simulink model "dcsim_shelf"  (R2026a)
settings: Solver=ode23t  StopTime=7e-3  MaxStep=1e-6  RelTol=1e-6  AbsTol=1e-6
values from neighbouring files (symbols this model uses):
  prm = [shared.V_ref, shared.P_rated, shared.V_uvlo, c.smooth_on, shared.S_max, shared.tau_r,         shared.p_fix, shared.k2, shared.V_ref48, shared.K_p, shared.K_i, shared.tau_i, shared.I_lim_out,         shared.V_uvlo48, 1.0, shared.t_uvlo48, shared.V_hyst48]    [load_case.m]
undefined symbols (not defined in the file or in its folder): ic_i_co, ic_P_cmd, ic_v_c, ic_v_Cin, ic_v_out, ic_xi_v, R_droop, R_esr, R_f, R_f48, R_in, R_in_esr, R_line, R_out_esr, t_event, tau_c, tau_sense, V_ref
libraries: fl_lib x31, nesl_utility x13
Description:
  | dcsim_shelf build 2026-09-18h (control states integrated explicitly at 1 us in ctrl_d)
settings Model: Creator=USER  LastModifiedBy=USER

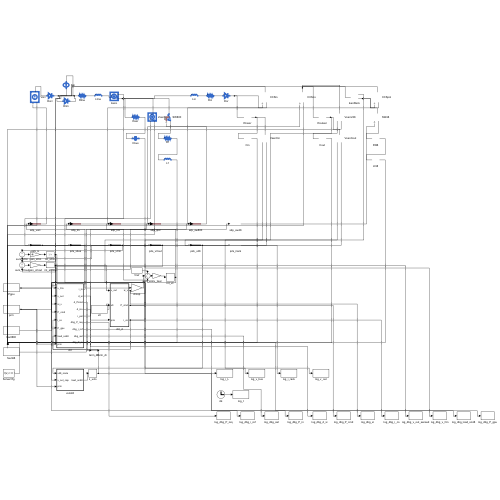
[thumbnail: Simulink's stored preview of the top-level diagram]
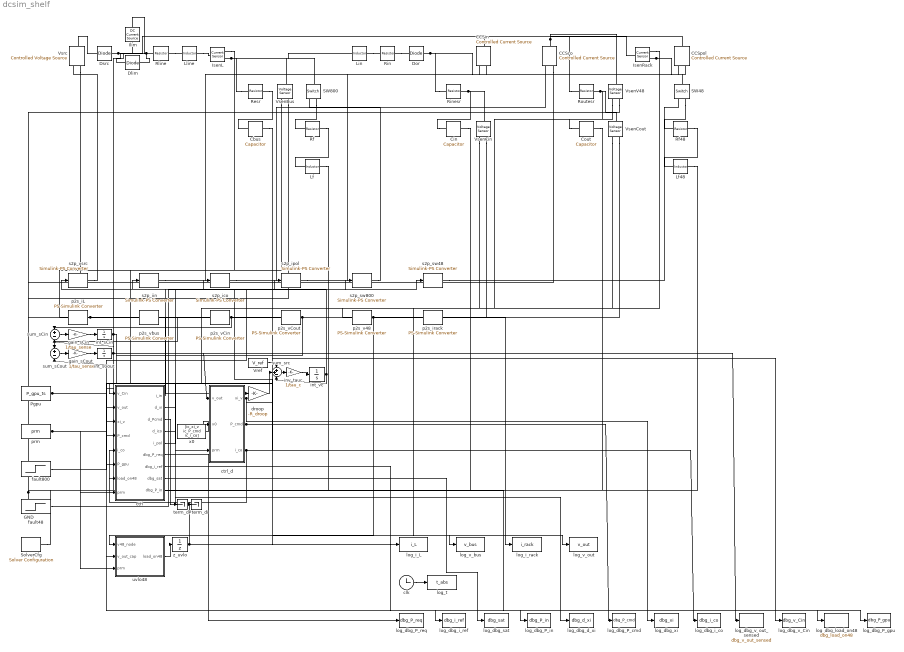
== system dcsim_shelf ==
  CCSco : fl_lib/Electrical/Electrical Sources/Controlled Current Source
  CCSin : fl_lib/Electrical/Electrical Sources/Controlled Current Source
  CCSpol : fl_lib/Electrical/Electrical Sources/Controlled Current Source
  Cbus : fl_lib/Electrical/Electrical Elements/Capacitor  c=C_bus F  r=1e-6 Ohm  g=0 1/Ohm  i_specify=off  i_priority=None  i=0 A  i_nominal_specify=off  i_nominal_value=1  i_nominal_unit=A  v_specify=off  v_priority=None  v=0 V  v_nominal_specify=off  v_nominal_value=1  v_nominal_unit=V  vc_specify=on  vc_priority=High  vc=ic_v_C V  vc_nominal_specify=off  vc_nominal_value=1  vc_nominal_unit=V
  Cin : fl_lib/Electrical/Electrical Elements/Capacitor  c=C_in F  r=1e-6 Ohm  g=0 1/Ohm  i_specify=off  i_priority=None  i=0 A  i_nominal_specify=off  i_nominal_value=1  i_nominal_unit=A  v_specify=off  v_priority=None  v=0 V  v_nominal_specify=off  v_nominal_value=1  v_nominal_unit=V  vc_specify=on  vc_priority=High  vc=ic_v_Cin V  vc_nominal_specify=off  vc_nominal_value=1  vc_nominal_unit=V
  Cout : fl_lib/Electrical/Electrical Elements/Capacitor  c=C_out F  r=1e-6 Ohm  g=0 1/Ohm  i_specify=off  i_priority=None  i=0 A  i_nominal_specify=off  i_nominal_value=1  i_nominal_unit=A  v_specify=off  v_priority=None  v=0 V  v_nominal_specify=off  v_nominal_value=1  v_nominal_unit=V  vc_specify=on  vc_priority=High  vc=ic_v_out V  vc_nominal_specify=off  vc_nominal_value=1  vc_nominal_unit=V
  Dlim : fl_lib/Electrical/Electrical Elements/Diode  Vf=1e-9 V  Ron=1e-6 Ohm  Goff=1e-8 1/Ohm  i_specify=off  i_priority=None  i=0 A  i_nominal_specify=off  i_nominal_value=1  i_nominal_unit=A  v_specify=off  v_priority=None  v=0 V  v_nominal_specify=off  v_nominal_value=1  v_nominal_unit=V
  Dor : fl_lib/Electrical/Electrical Elements/Diode  Vf=1e-9 V  Ron=1e-6 Ohm  Goff=1e-8 1/Ohm  i_specify=off  i_priority=None  i=0 A  i_nominal_specify=off  i_nominal_value=1  i_nominal_unit=A  v_specify=off  v_priority=None  v=0 V  v_nominal_specify=off  v_nominal_value=1  v_nominal_unit=V
  Dsrc : fl_lib/Electrical/Electrical Elements/Diode  Vf=1e-9 V  Ron=1e-6 Ohm  Goff=1e-8 1/Ohm  i_specify=off  i_priority=None  i=0 A  i_nominal_specify=off  i_nominal_value=1  i_nominal_unit=A  v_specify=off  v_priority=None  v=0 V  v_nominal_specify=off  v_nominal_value=1  v_nominal_unit=V
  GND : fl_lib/Electrical/Electrical Elements/Electrical Reference
  Ilim : fl_lib/Electrical/Electrical Sources/DC Current Source  i0=I_lim A
  IsenL : fl_lib/Electrical/Electrical Sensors/Current Sensor
  IsenRack : fl_lib/Electrical/Electrical Sensors/Current Sensor
  Lf : fl_lib/Electrical/Electrical Elements/Inductor  l=L_f H  r=0 Ohm  g=1e-9 1/Ohm  i_specify=off  i_priority=None  i=0 A  i_nominal_specify=off  i_nominal_value=1  i_nominal_unit=A  v_specify=off  v_priority=None  v=0 V  v_nominal_specify=off  v_nominal_value=1  v_nominal_unit=V  i_L_specify=on  i_L_priority=High  i_L=0 A  i_L_nominal_specify=off  i_L_nominal_value=1  i_L_nominal_unit=A
  Lf48 : fl_lib/Electrical/Electrical Elements/Inductor  l=L_f48 H  r=0 Ohm  g=1e-9 1/Ohm  i_specify=off  i_priority=None  i=0 A  i_nominal_specify=off  i_nominal_value=1  i_nominal_unit=A  v_specify=off  v_priority=None  v=0 V  v_nominal_specify=off  v_nominal_value=1  v_nominal_unit=V  i_L_specify=on  i_L_priority=High  i_L=0 A  i_L_nominal_specify=off  i_L_nominal_value=1  i_L_nominal_unit=A
  Lin : fl_lib/Electrical/Electrical Elements/Inductor  l=L_in H  r=0 Ohm  g=1e-9 1/Ohm  i_specify=off  i_priority=None  i=0 A  i_nominal_specify=off  i_nominal_value=1  i_nominal_unit=A  v_specify=off  v_priority=None  v=0 V  v_nominal_specify=off  v_nominal_value=1  v_nominal_unit=V  i_L_specify=on  i_L_priority=High  i_L=ic_i_Lin A  i_L_nominal_specify=off  i_L_nominal_value=1  i_L_nominal_unit=A
  Lline : fl_lib/Electrical/Electrical Elements/Inductor  l=L_line H  r=0 Ohm  g=1e-9 1/Ohm  i_specify=off  i_priority=None  i=0 A  i_nominal_specify=off  i_nominal_value=1  i_nominal_unit=A  v_specify=off  v_priority=None  v=0 V  v_nominal_specify=off  v_nominal_value=1  v_nominal_unit=V  i_L_specify=on  i_L_priority=High  i_L=ic_i_L A  i_L_nominal_specify=off  i_L_nominal_value=1  i_L_nominal_unit=A
  Pgpu : FromWorkspace  VariableName=P_gpu_ts
  Resr : fl_lib/Electrical/Electrical Elements/Resistor  R=R_esr - 1e-6 Ohm  i_specify=off  i_priority=None  i=0 A  i_nominal_specify=off  i_nominal_value=1  i_nominal_unit=A  v_specify=off  v_priority=None  v=0 V  v_nominal_specify=off  v_nominal_value=1  v_nominal_unit=V
  Rf : fl_lib/Electrical/Electrical Elements/Resistor  R=R_f - 1e-6 Ohm  i_specify=off  i_priority=None  i=0 A  i_nominal_specify=off  i_nominal_value=1  i_nominal_unit=A  v_specify=off  v_priority=None  v=0 V  v_nominal_specify=off  v_nominal_value=1  v_nominal_unit=V
  Rf48 : fl_lib/Electrical/Electrical Elements/Resistor  R=R_f48 - 1e-6 Ohm  i_specify=off  i_priority=None  i=0 A  i_nominal_specify=off  i_nominal_value=1  i_nominal_unit=A  v_specify=off  v_priority=None  v=0 V  v_nominal_specify=off  v_nominal_value=1  v_nominal_unit=V
  Rin : fl_lib/Electrical/Electrical Elements/Resistor  R=R_in Ohm  i_specify=off  i_priority=None  i=0 A  i_nominal_specify=off  i_nominal_value=1  i_nominal_unit=A  v_specify=off  v_priority=None  v=0 V  v_nominal_specify=off  v_nominal_value=1  v_nominal_unit=V
  Rinesr : fl_lib/Electrical/Electrical Elements/Resistor  R=R_in_esr - 1e-6 Ohm  i_specify=off  i_priority=None  i=0 A  i_nominal_specify=off  i_nominal_value=1  i_nominal_unit=A  v_specify=off  v_priority=None  v=0 V  v_nominal_specify=off  v_nominal_value=1  v_nominal_unit=V
  Rline : fl_lib/Electrical/Electrical Elements/Resistor  R=R_line Ohm  i_specify=off  i_priority=None  i=0 A  i_nominal_specify=off  i_nominal_value=1  i_nominal_unit=A  v_specify=off  v_priority=None  v=0 V  v_nominal_specify=off  v_nominal_value=1  v_nominal_unit=V
  Routesr : fl_lib/Electrical/Electrical Elements/Resistor  R=R_out_esr - 1e-6 Ohm  i_specify=off  i_priority=None  i=0 A  i_nominal_specify=off  i_nominal_value=1  i_nominal_unit=A  v_specify=off  v_priority=None  v=0 V  v_nominal_specify=off  v_nominal_value=1  v_nominal_unit=V
  SW48 : fl_lib/Electrical/Electrical Elements/Switch  R_closed=1e-6 Ohm  G_open=1e-8 1/Ohm  Threshold=0.5  i_specify=off  i_priority=None  i=0 A  i_nominal_specify=off  i_nominal_value=1  i_nominal_unit=A  v_specify=off  v_priority=None  v=0 V  v_nominal_specify=off  v_nominal_value=1  v_nominal_unit=V
  SW800 : fl_lib/Electrical/Electrical Elements/Switch  R_closed=1e-6 Ohm  G_open=1e-8 1/Ohm  Threshold=0.5  i_specify=off  i_priority=None  i=0 A  i_nominal_specify=off  i_nominal_value=1  i_nominal_unit=A  v_specify=off  v_priority=None  v=0 V  v_nominal_specify=off  v_nominal_value=1  v_nominal_unit=V
  SolverCfg : nesl_utility/Solver Configuration  PhysicalDomain=network_engine_domain  SubClassName=solver  LeftPortType=input  RightPortType=generic  Tones=[]  Harmonics=[]  SimulateNoise=off  Profile=off  UseLocalSampling=off  EnableSwitchedLinearOptims=on  FrequencyDomain=off  UseCCode=off  RelTol=0.001  AbsTol=0.001  MinStep=1e-09  ToWorkspace=off  RevertToSquareIcSolve=off  NumHomotopyIterations=100  PhasorMode=off  PhasorModeNumHarmonics=1  ConsistencySolver=NEWTON_XTOL_AFTER_FTOL  CanonicalOrdering=CANONICAL  OptimizeIntermediates=OPTIMIZED  IndexReductionMethod=DerivativeReplacement  DoDC=off  ResidualTolerance=1e-09  ConsistencyTolSource=GLOBAL  ConsistencyAbsTol=0.001  ConsistencyRelTol=0.001  ConsistencyTolFactor=0.001  UseLocalSolver=off  LocalSolverChoice=NE_BACKWARD_EULER_ADVANCER  ResolveIndetEquations=on  FunctionEvalNumThread=1  LocalSolverSampleTime=0.001  DoFixedCost=off  MaxNonlinIter=3  MaxModeIter=2  ComputeImpulses=off  ImpulseIterations=2  LinearAlgebra=auto  LinearAlgebraNumThread=0  EquationFormulation=NE_TIME_EF  DelaysMemoryBudget=1024  AutomaticFiltering=on  FilteringTimeConstant=0.001  PartitionStorageMethod=AS_NEEDED  PartitionMemoryBudget=1024  PartitionMethod=ROBUST  MultibodyUseLocalSolver=off  MultibodyLocalSolverChoice=ODE1  MultibodyLocalSolverSampleTime=0.001
  Vref : Constant  Value=V_ref
  VsenBus : fl_lib/Electrical/Electrical Sensors/Voltage Sensor
  VsenCin : fl_lib/Electrical/Electrical Sensors/Voltage Sensor
  VsenCout : fl_lib/Electrical/Electrical Sensors/Voltage Sensor
  VsenV48 : fl_lib/Electrical/Electrical Sensors/Voltage Sensor
  Vsrc : fl_lib/Electrical/Electrical Sources/Controlled Voltage Source
  clk : Clock
  ctrl : MATLAB Function  TreatAsAtomicUnit=on
  ctrl_d : MATLAB Function  TreatAsAtomicUnit=on
  droop : Gain  Gain=-R_droop
  fault48 : Step  Time=t_event  FinalValue=f48_on  SampleTime=0
  fault800 : Step  Time=t_event  FinalValue=f800_on  SampleTime=0
  gain_sCin : Gain  Gain=1/tau_sense
  gain_sCout : Gain  Gain=1/tau_sense
  int_sCin : Integrator  InitialCondition=ic_v_Cin
  int_sCout : Integrator  InitialCondition=ic_v_out
  int_vc : Integrator  InitialCondition=ic_v_c
  inv_tauc : Gain  Gain=1/tau_c
  log_dbg_P_cmd : ToWorkspace  VariableName=dbg_P_cmd  SampleTime=-1
  log_dbg_P_gpu : ToWorkspace  VariableName=dbg_P_gpu  SampleTime=-1
  log_dbg_P_in : ToWorkspace  VariableName=dbg_P_in  SampleTime=-1
  log_dbg_P_req : ToWorkspace  VariableName=dbg_P_req  SampleTime=-1
  log_dbg_d_xi : ToWorkspace  VariableName=dbg_d_xi  SampleTime=-1
  log_dbg_i_co : ToWorkspace  VariableName=dbg_i_co  SampleTime=-1
  log_dbg_i_ref : ToWorkspace  VariableName=dbg_i_ref  SampleTime=-1
  log_dbg_load_on48 : ToWorkspace  VariableName=dbg_load_on48  SampleTime=-1
  log_dbg_sat : ToWorkspace  VariableName=dbg_sat  SampleTime=-1
  log_dbg_v_Cin : ToWorkspace  VariableName=dbg_v_Cin  SampleTime=-1
  log_dbg_v_out_sensed : ToWorkspace  VariableName=dbg_v_out_sensed  SampleTime=-1
  log_dbg_xi : ToWorkspace  VariableName=dbg_xi  SampleTime=-1
  log_i_L : ToWorkspace  VariableName=i_L  SampleTime=-1
  log_i_rack : ToWorkspace  VariableName=i_rack  SampleTime=-1
  log_t : ToWorkspace  VariableName=t_abs  SampleTime=-1
  log_v_bus : ToWorkspace  VariableName=v_bus  SampleTime=-1
  log_v_out : ToWorkspace  VariableName=v_out  SampleTime=-1
  p2s_iL : nesl_utility/PS-Simulink Converter  PhysicalDomain=network_engine_domain  SubClassName=ps_output  LeftPortType=input  RightPortType=output  PseudoPeriodic=off  Frequencies=[]  VectorFormat=inherit  Unit=inherit  AffineConversion=off
  p2s_irack : nesl_utility/PS-Simulink Converter  PhysicalDomain=network_engine_domain  SubClassName=ps_output  LeftPortType=input  RightPortType=output  PseudoPeriodic=off  Frequencies=[]  VectorFormat=inherit  Unit=inherit  AffineConversion=off
  p2s_v48 : nesl_utility/PS-Simulink Converter  PhysicalDomain=network_engine_domain  SubClassName=ps_output  LeftPortType=input  RightPortType=output  PseudoPeriodic=off  Frequencies=[]  VectorFormat=inherit  Unit=inherit  AffineConversion=off
  p2s_vCin : nesl_utility/PS-Simulink Converter  PhysicalDomain=network_engine_domain  SubClassName=ps_output  LeftPortType=input  RightPortType=output  PseudoPeriodic=off  Frequencies=[]  VectorFormat=inherit  Unit=inherit  AffineConversion=off
  p2s_vCout : nesl_utility/PS-Simulink Converter  PhysicalDomain=network_engine_domain  SubClassName=ps_output  LeftPortType=input  RightPortType=output  PseudoPeriodic=off  Frequencies=[]  VectorFormat=inherit  Unit=inherit  AffineConversion=off
  p2s_vbus : nesl_utility/PS-Simulink Converter  PhysicalDomain=network_engine_domain  SubClassName=ps_output  LeftPortType=input  RightPortType=output  PseudoPeriodic=off  Frequencies=[]  VectorFormat=inherit  Unit=inherit  AffineConversion=off
  prm : Constant  Value=prm
  s2p_ico : nesl_utility/Simulink-PS Converter  PhysicalDomain=network_engine_domain  SubClassName=ps_input  LeftPortType=input  RightPortType=output  PseudoPeriodic=off  Frequencies=[]  NoiseDistribution=none  NoiseParameters=[]  Unit=1  AffineConversion=off  FilteringAndDerivatives=provide  SimscapeFilterOrder=1  InputFilterTimeConstant=0.001  UdotUserProvided=0
  s2p_iin : nesl_utility/Simulink-PS Converter  PhysicalDomain=network_engine_domain  SubClassName=ps_input  LeftPortType=input  RightPortType=output  PseudoPeriodic=off  Frequencies=[]  NoiseDistribution=none  NoiseParameters=[]  Unit=1  AffineConversion=off  FilteringAndDerivatives=provide  SimscapeFilterOrder=1  InputFilterTimeConstant=0.001  UdotUserProvided=0
  s2p_ipol : nesl_utility/Simulink-PS Converter  PhysicalDomain=network_engine_domain  SubClassName=ps_input  LeftPortType=input  RightPortType=output  PseudoPeriodic=off  Frequencies=[]  NoiseDistribution=none  NoiseParameters=[]  Unit=1  AffineConversion=off  FilteringAndDerivatives=provide  SimscapeFilterOrder=1  InputFilterTimeConstant=0.001  UdotUserProvided=0
  s2p_sw48 : nesl_utility/Simulink-PS Converter  PhysicalDomain=network_engine_domain  SubClassName=ps_input  LeftPortType=input  RightPortType=output  PseudoPeriodic=off  Frequencies=[]  NoiseDistribution=none  NoiseParameters=[]  Unit=1  AffineConversion=off  FilteringAndDerivatives=provide  SimscapeFilterOrder=1  InputFilterTimeConstant=0.001  UdotUserProvided=0
  s2p_sw800 : nesl_utility/Simulink-PS Converter  PhysicalDomain=network_engine_domain  SubClassName=ps_input  LeftPortType=input  RightPortType=output  PseudoPeriodic=off  Frequencies=[]  NoiseDistribution=none  NoiseParameters=[]  Unit=1  AffineConversion=off  FilteringAndDerivatives=provide  SimscapeFilterOrder=1  InputFilterTimeConstant=0.001  UdotUserProvided=0
  s2p_vsrc : nesl_utility/Simulink-PS Converter  PhysicalDomain=network_engine_domain  SubClassName=ps_input  LeftPortType=input  RightPortType=output  PseudoPeriodic=off  Frequencies=[]  NoiseDistribution=none  NoiseParameters=[]  Unit=1  AffineConversion=off  FilteringAndDerivatives=provide  SimscapeFilterOrder=1  InputFilterTimeConstant=0.001  UdotUserProvided=0
  sum_sCin : Sum  Inputs=+-
  sum_sCout : Sum  Inputs=+-
  sum_src : Sum  Inputs=++-
  term_dP : Terminator
  term_di : Terminator
  uvlo48 : MATLAB Function  TreatAsAtomicUnit=on
  x0 : Constant  Value=[ic_xi_v ic_P_cmd ic_i_co]
  z_uvlo : UnitDelay  InitialCondition=1  SampleTime=1e-6
  wires:
  p2s_vCin/1 -> sum_sCin/1, log_dbg_v_Cin/1
  int_sCin/1 -> sum_sCin/2, ctrl/1(v_Cin)
  sum_sCin/1 -> gain_sCin/1
  gain_sCin/1 -> int_sCin/1
  p2s_vCout/1 -> sum_sCout/1, uvlo48/2(v_out_cap)
  int_sCout/1 -> sum_sCout/2, ctrl/2(v_out), ctrl_d/1(v_out), log_dbg_v_out_sensed/1
  sum_sCout/1 -> gain_sCout/1
  gain_sCout/1 -> int_sCout/1
  x0/1 -> ctrl_d/2(x0)
  prm/1 -> ctrl_d/3(prm), ctrl/8(prm), uvlo48/3(prm)
  ctrl_d/1(xi_v) -> ctrl/3(xi_v), log_dbg_xi/1
  ctrl_d/2(P_cmd) -> ctrl/4(P_cmd), log_dbg_P_cmd/1
  ctrl_d/3(i_co) -> ctrl/5(i_co), s2p_ico/1, log_dbg_i_co/1
  Pgpu/1 -> ctrl/6(P_gpu), log_dbg_P_gpu/1
  uvlo48/1(load_on48) -> z_uvlo/1
  z_uvlo/1 -> ctrl/7(load_on48), log_dbg_load_on48/1
  ctrl/1(i_in) -> s2p_iin/1
  ctrl/5(i_pol) -> s2p_ipol/1
  ctrl/3(d_Pcmd) -> term_dP/1
  ctrl/4(d_ico) -> term_di/1
  p2s_v48/1 -> uvlo48/1(v48_node), log_v_out/1
  p2s_iL/1 -> droop/1, log_i_L/1
  droop/1 -> sum_src/2
  Vref/1 -> sum_src/1
  int_vc/1 -> sum_src/3, s2p_vsrc/1
  sum_src/1 -> inv_tauc/1
  inv_tauc/1 -> int_vc/1
  fault800/1 -> s2p_sw800/1
  fault48/1 -> s2p_sw48/1
  p2s_vbus/1 -> log_v_bus/1
  p2s_irack/1 -> log_i_rack/1
  clk/1 -> log_t/1
  ctrl/6(dbg_P_req) -> log_dbg_P_req/1
  ctrl/7(dbg_i_ref) -> log_dbg_i_ref/1
  ctrl/8(dbg_sat) -> log_dbg_sat/1
  ctrl/9(dbg_P_in) -> log_dbg_P_in/1
  ctrl/2(d_xi) -> log_dbg_d_xi/1
  connections:
  SolverCfg/RConn1 -- Vsrc/RConn2 -- Cbus/RConn1 -- VsenBus/RConn2 -- Lf/RConn1 -- Cin/RConn1 -- VsenCin/RConn2 -- CCSin/LConn1 -- CCSco/RConn2 -- Cout/RConn1 -- VsenCout/RConn2 -- VsenV48/RConn2 -- CCSpol/LConn1 -- GND/LConn1 -- Lf48/RConn1
  Vsrc/LConn1 -- Dsrc/LConn1
  Ilim/RConn1 -- Dsrc/RConn1 -- Dlim/RConn1
  Rline/LConn1 -- Ilim/LConn1 -- Dlim/LConn1
  Rline/RConn1 -- Lline/LConn1
  Lline/RConn1 -- IsenL/LConn1
  Resr/LConn1 -- IsenL/RConn2 -- VsenBus/LConn1 -- SW800/LConn1 -- Lin/LConn1
  Resr/RConn1 -- Cbus/LConn1
  SW800/RConn2 -- Rf/LConn1
  Rf/RConn1 -- Lf/LConn1
  Lin/RConn1 -- Rin/LConn1
  Rin/RConn1 -- Dor/LConn1
  Rinesr/LConn1 -- Dor/RConn1 -- CCSin/RConn2
  Cin/LConn1 -- Rinesr/RConn1 -- VsenCin/LConn1
  Routesr/LConn1 -- CCSco/LConn1 -- VsenV48/LConn1 -- IsenRack/LConn1
  Cout/LConn1 -- Routesr/RConn1 -- VsenCout/LConn1
  CCSpol/RConn2 -- IsenRack/RConn2 -- SW48/LConn1
  SW48/RConn2 -- Rf48/LConn1
  Rf48/RConn1 -- Lf48/LConn1
  s2p_vsrc/RConn1 -- Vsrc/RConn1
  s2p_iin/RConn1 -- CCSin/RConn1
  s2p_ico/RConn1 -- CCSco/RConn1
  s2p_ipol/RConn1 -- CCSpol/RConn1
  s2p_sw800/RConn1 -- SW800/RConn1
  s2p_sw48/RConn1 -- SW48/RConn1
  IsenL/RConn1 -- p2s_iL/LConn1
  VsenBus/RConn1 -- p2s_vbus/LConn1
  VsenCin/RConn1 -- p2s_vCin/LConn1
  VsenCout/RConn1 -- p2s_vCout/LConn1
  VsenV48/RConn1 -- p2s_v48/LConn1
  IsenRack/RConn1 -- p2s_irack/LConn1

== matlab function dcsim_shelf/ctrl ==
  data: v_Cin input; i_in output; v_out input; xi_v input; P_cmd input; i_co input; P_gpu input; load_on48 input; prm input; d_xi output; d_Pcmd output; d_ico output; i_pol output; dbg_P_req output; dbg_i_ref output; dbg_sat output; dbg_P_in output
function [i_in, d_xi, d_Pcmd, d_ico, i_pol, dbg_P_req, dbg_i_ref, dbg_sat, dbg_P_in] = ctrl(v_Cin, v_out, xi_v, P_cmd, i_co, P_gpu, load_on48, prm)
% One-to-one with dcsim/model_v04.py _derivs (control part). Pure algebra;
% the three integrators live outside. v_Cin and v_out are CAPACITOR voltages.
V_ref=prm(1); P_rated=prm(2); V_uvlo=prm(3); smooth_on=prm(4); S_max=prm(5); tau_r=prm(6);
p_fix=prm(7); k2=prm(8); V_ref48=prm(9); K_p=prm(10); K_i=prm(11); tau_i=prm(12); I_lim_out=prm(13);
V_uvlo48=prm(14); conv_on=prm(15);
% ---- POL load (48 V constant power with UVLO floor)
i_pol = 0;
if load_on48 > 0.5, i_pol = P_gpu / max(v_out, V_uvlo48); end
% ---- voltage loop demand
err = V_ref48 - v_out;
i_ref = K_p*err + K_i*xi_v;
sat = min(max(i_ref, 0), I_lim_out);
P_out_dem = max(v_out*sat, 0);
P_req = 0; if conv_on > 0.5, P_req = P_out_dem + p_fix*P_rated + k2*P_out_dem^2/P_rated; end
% ---- converter-input ramp limiter (one state: P_cmd)
d_Pcmd = 0; P_in = P_req;
if smooth_on > 0.5
    d_Pcmd = min(max((P_req - P_cmd)/tau_r, -S_max), S_max);
    if conv_on > 0.5, P_in = P_cmd; else, P_in = 0; end
    P_out_max = max(P_in - p_fix*P_rated, 0);
    i_co_max = P_out_max / max(v_out, 1);
    if sat > i_co_max, sat = i_co_max; end
end
% ---- anti-windup: freeze whenever the FINAL command differs from i_ref (no sign test)
if sat == i_ref, d_xi = err; else, d_xi = 0; end
% ---- inner current loop
if conv_on > 0.5, d_ico = (sat - i_co)/tau_i; else, d_ico = -i_co/tau_i; end
% ---- converter input draw from the input capacitor
i_in = 0; if conv_on > 0.5, i_in = P_in / max(v_Cin, V_uvlo); end
% ---- diagnostics only (logged, never fed back)
dbg_P_req = P_req; dbg_i_ref = i_ref; dbg_sat = sat; dbg_P_in = P_in;
end

== matlab function dcsim_shelf/ctrl_d ==
  settings: updateMethod=DISCRETE  sampleTime=1e-6
  data: v_out input; xi_v output; x0 input; prm input; P_cmd output; i_co output
function [xi_v, P_cmd, i_co] = ctrl_d(v_out, x0, prm)
% Explicit RK4 at Ts = 1 us for the three control states, v_out (sensed capacitor voltage) held over the step.
% Same right-hand side as dcsim/model_v04.py _derivs (states 7, 6, 8) and as the diagnostic outputs of ctrl.
persistent x
if isempty(x), x = [x0(1); x0(2); x0(3)]; end
xi_v = x(1); P_cmd = x(2); i_co = x(3);
h = 1e-6;
k1 = rhs(x, v_out, prm);
k2 = rhs(x + 0.5*h*k1, v_out, prm);
k3 = rhs(x + 0.5*h*k2, v_out, prm);
k4 = rhs(x + h*k3, v_out, prm);
x = x + (h/6)*(k1 + 2*k2 + 2*k3 + k4);
end
function dx = rhs(x, v_out, prm)
P_rated=prm(2); smooth_on=prm(4); S_max=prm(5); tau_r=prm(6); p_fix=prm(7); k2c=prm(8);
V_ref48=prm(9); K_p=prm(10); K_i=prm(11); tau_i=prm(12); I_lim_out=prm(13); conv_on=prm(15);
xi_v = x(1); P_cmd = x(2); i_co = x(3);
err = V_ref48 - v_out;
i_ref = K_p*err + K_i*xi_v;
sat = min(max(i_ref, 0), I_lim_out);
P_out_dem = max(v_out*sat, 0);
P_req = 0; if conv_on > 0.5, P_req = P_out_dem + p_fix*P_rated + k2c*P_out_dem^2/P_rated; end
d_Pcmd = 0;
if smooth_on > 0.5
    d_Pcmd = min(max((P_req - P_cmd)/tau_r, -S_max), S_max);
    P_in = 0; if conv_on > 0.5, P_in = P_cmd; end
    i_co_max = max(P_in - p_fix*P_rated, 0) / max(v_out, 1);
    if sat > i_co_max, sat = i_co_max; end
end
d_xi = 0; if sat == i_ref, d_xi = err; end
if conv_on > 0.5, d_ico = (sat - i_co)/tau_i; else, d_ico = -i_co/tau_i; end
dx = [d_xi; d_Pcmd; d_ico];
end

== matlab function dcsim_shelf/uvlo48 ==
  settings: updateMethod=DISCRETE  sampleTime=1e-6
  data: v48_node input; load_on48 output; v_out_cap input; prm input
function load_on48 = uvlo48(v48_node, v_out_cap, prm)
% POL UVLO state machine, sampled at 1 us (block Sample time). Compares the
% NODE voltage (with ESR) for the trip, the CAPACITOR voltage for recovery,
% as dcsim/model_v04.py simulate() does.
V_ref48=prm(9); V_uvlo48=prm(14); t_uvlo48=prm(16); V_hyst48=prm(17); Ts=1e-6;
persistent tmr on
if isempty(tmr), tmr = 0; on = true; end
if v48_node < V_uvlo48
    tmr = tmr + Ts;
    if tmr >= t_uvlo48, on = false; end
else
    tmr = 0;
    if ~on && v_out_cap > V_uvlo48 + V_hyst48, on = true; end
end
load_on48 = double(on);
end
